simulink model "basicModel_old"  (R2017b)
settings: Solver=ode3  StartTime=0.0  StopTime=40  FixedStep=0.01  RelTol=1e-3  EnableMultiTasking=on
InitFcn:
  | clear;
  | clc;
  | Iniparameters
StopFcn:
  | simplot
values from neighbouring files (symbols this model uses):
  aaa = inv([kf kf kf kf;0 -kf 0 kf;-kf 0 kf 0;-km km -km km])    [Iniparameters.m]
  g = 9.8    [Iniparameters.m]
  Ixx = 19.688e-3    (= 0.019688)    [Iniparameters.m]
  Iyy = 19.688e-3    (= 0.019688)    [Iniparameters.m]
  Izz = 3.938e-2    (= 0.03938)    [Iniparameters.m]
  kdphi = 8    [Iniparameters.m]
  kdpsai = 8    [Iniparameters.m]
  kdtheta = kdphi    (= 8)    [Iniparameters.m]
  kdx = 0.55    [Iniparameters.m]
  kdy = 2.0    (= 2)    [Iniparameters.m]
  kdz = 2.4    [Iniparameters.m]
  kf = 3.13e-5    (= 3.13e-05)    [Iniparameters.m]
  kix = 0.001    [Iniparameters.m]
  kiy = 0.001    [Iniparameters.m]
  kiz = 0.001    [Iniparameters.m]
  km = 7.5e-7    (= 7.5e-07)    [Iniparameters.m]
  kpphi = 25    [Iniparameters.m]
  kppsai = 23    [Iniparameters.m]
  kptheta = kpphi    (= 25)    [Iniparameters.m]
  kpx = 0.75    [Iniparameters.m]
  kpy = 1.4    [Iniparameters.m]
  kpz = 2.9    [Iniparameters.m]
  L = 0.25    [Iniparameters.m]
  m = 0.75    [Iniparameters.m]
  wh = sqrt(m*g/(4*kf))    [Iniparameters.m]
  xf = 5    [Iniparameters.m]
  yaw = 0    [Iniparameters.m]
  yf = 5    [Iniparameters.m]
  zf = 5    [Iniparameters.m]
libraries: aerolibconvert2 x4
settings Model: Creator=KingBoy  LastModifiedBy=KingBoy
settings DataIOCC: LimitDataPoints=on  SaveFormat=Array
settings OptimizationCC: LifeSpan=inf
settings DebuggingCC: UnderspecifiedInitializationDetection=Classic  MergeDetectMultiDrivingBlocksExec=none  SolverPrmCheckMsg=warning  AllowSymbolicDim=off  SFUnexpectedBacktrackingDiag=warning  SFNoUnconditionalDefaultTransitionDiag=warning  SFExecutionAtInitializationDiag=none
settings HardwareCC: ProdBitPerPointer=32  ProdBitPerSizeT=32  ProdBitPerPtrDiffT=32  ProdLargestAtomicFloat=None  ProdIntDivRoundTo=Undefined  ProdEndianess=Unspecified  ProdWordSize=32  ProdHWDeviceType=32-bit Generic
settings ModelReferenceCC: PropagateSignalLabelsOutOfModel=off
settings CodeAppCC: StateflowObjectComments=on
settings GRTTargetCC: TargetLangStandard=C89/C90 (ANSI)  GeneratePreprocessorConditionals=Disable all
settings ConfigComp: CovMetricSettings=dw  CovHtmlReporting=on  CovSaveCumulativeToWorkspaceVar=on  CovSaveSingleToWorkspaceVar=on  CovExternalEMLEnable=off  CovSFcnEnable=off

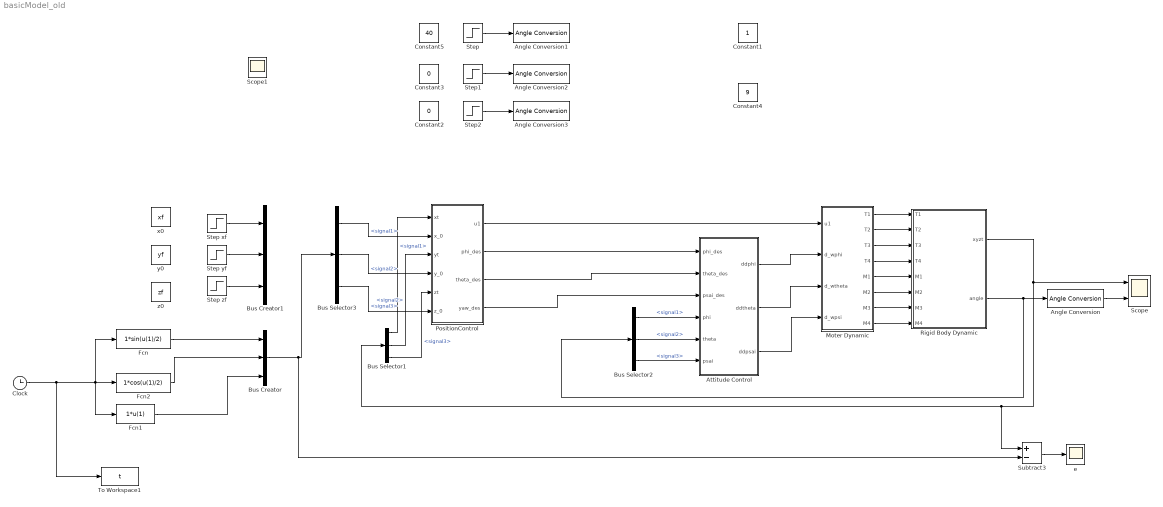
== system basicModel_old ==
  Angle Conversion : aerolibconvert2/Angle Conversion  IU=rad  OU=deg
  Angle Conversion1 : aerolibconvert2/Angle Conversion  IU=deg  OU=rad
  Angle Conversion2 : aerolibconvert2/Angle Conversion  IU=deg  OU=rad
  Angle Conversion3 : aerolibconvert2/Angle Conversion  IU=deg  OU=rad
  Attitude Control : Subsystem
  Bus Creator : BusCreator  Inputs=3
  Bus Creator1 : BusCreator  Inputs=3
  Bus Selector1 : BusSelector  OutputSignals=signal1,signal2,signal3
  Bus Selector2 : BusSelector  OutputSignals=signal1,signal2,signal3
  Bus Selector3 : BusSelector  OutputSignals=signal1,signal2,signal3
  Clock : Clock
  Constant1 : Constant
  Constant2 : Constant  Value=0
  Constant3 : Constant  Value=0
  Constant4 : Constant  Value=9
  Constant5 : Constant  Value=40
  Fcn : Fcn  Expr=1*sin(u(1)/2)
  Fcn1 : Fcn  Expr=1*u(1)
  Fcn2 : Fcn  Expr=1*cos(u(1)/2)
  Moter Dynamic : Subsystem
  PositionControl : Subsystem
  Rigid Body Dynamic : Subsystem
  Scope : Scope  NumInputPorts=2
  Scope1 : Scope
  Step : Step  After=xf  SampleTime=0
  Step xf : Step  After=xf  SampleTime=0
  Step yf : Step  After=yf  SampleTime=0
  Step zf : Step  After=zf  SampleTime=0
  Step1 : Step  After=yf  SampleTime=0
  Step2 : Step  After=zf  SampleTime=0
  Subtract3 : Sum  Inputs=+-
  To Workspace1 : ToWorkspace  VariableName=t  SampleTime=-1
      settings: Save2DSignal=2-D array (concatenate along first dimension)
  e : Scope
  x0 : Constant  Value=xf
  y0 : Constant  Value=yf
  z0 : Constant  Value=zf
  wires:
  Moter Dynamic/1(T1) -> Rigid Body Dynamic/1(T1)
  Moter Dynamic/2(T2) -> Rigid Body Dynamic/2(T2)
  Moter Dynamic/3(T3) -> Rigid Body Dynamic/3(T3)
  Moter Dynamic/4(T4) -> Rigid Body Dynamic/4(T4)
  Moter Dynamic/5(M1) -> Rigid Body Dynamic/5(M1)
  Moter Dynamic/6(M2) -> Rigid Body Dynamic/6(M2)
  Moter Dynamic/7(M3) -> Rigid Body Dynamic/7(M3)
  Moter Dynamic/8(M4) -> Rigid Body Dynamic/8(M4)
  Rigid Body Dynamic/1(xyzt) -> Subtract3/1, Bus Selector1/1, Scope/1
  Bus Selector1/1 -> PositionControl/1(xt)  "<signal1>"
  Bus Selector1/2 -> PositionControl/3(yt)  "<signal2>"
  Bus Selector1/3 -> PositionControl/5(zt)  "<signal3>"
  Rigid Body Dynamic/2(angle) -> Angle Conversion/1, Bus Selector2/1
  Angle Conversion/1 -> Scope/2
  Clock/1 -> To Workspace1/1, Fcn1/1, Fcn/1, Fcn2/1
  Fcn/1 -> Bus Creator/1
  Fcn2/1 -> Bus Creator/2
  Fcn1/1 -> Bus Creator/3
  Subtract3/1 -> e/1
  Bus Selector3/1 -> PositionControl/2(x_0)  "<signal1>"
  Bus Selector3/2 -> PositionControl/4(y_0)  "<signal2>"
  Bus Selector3/3 -> PositionControl/6(z_0)  "<signal3>"
  Step/1 -> Angle Conversion1/1
  Step2/1 -> Angle Conversion3/1
  Step1/1 -> Angle Conversion2/1
  Step zf/1 -> Bus Creator1/3
  Step yf/1 -> Bus Creator1/2
  Step xf/1 -> Bus Creator1/1
  Bus Selector2/3 -> Attitude Control/6(psai)  "<signal3>"
  Bus Selector2/2 -> Attitude Control/5(theta)  "<signal2>"
  Bus Selector2/1 -> Attitude Control/4(phi)  "<signal1>"
  Attitude Control/3(ddpsai) -> Moter Dynamic/4(d_wpsi)
  Attitude Control/2(ddtheta) -> Moter Dynamic/3(d_wtheta)
  Attitude Control/1(ddphi) -> Moter Dynamic/2(d_wphi)
  PositionControl/1(u1) -> Moter Dynamic/1(u1)
  PositionControl/2(phi_des) -> Attitude Control/1(phi_des)
  PositionControl/3(theta_des) -> Attitude Control/2(theta_des)
  PositionControl/4(yaw_des) -> Attitude Control/3(psai_des)
  Bus Creator/1 -> Subtract3/2, Bus Selector3/1

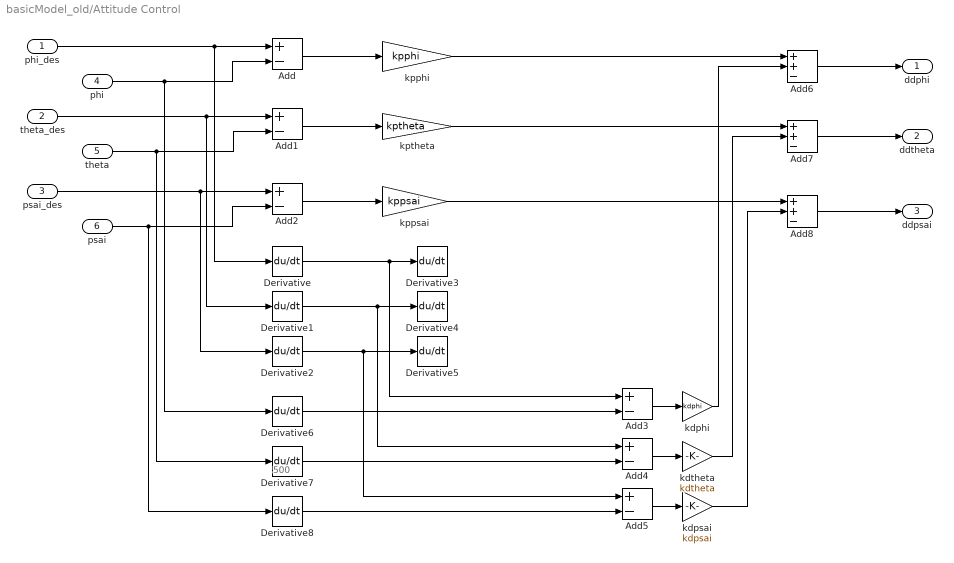
== system basicModel_old/Attitude Control ==
  note: 500
  phi_des : Inport
  theta_des : Inport  Port=2
  psai_des : Inport  Port=3
  phi : Inport  Port=4
  theta : Inport  Port=5
  psai : Inport  Port=6
  Add{,1..5} (6 alike) : Sum  Inputs=+-
  Add6 : Sum  Inputs=++-
  Add7 : Sum  Inputs=++-
  Add8 : Sum  Inputs=++-
  Derivative{,1..8} (9 alike) : Derivative  CoefficientInTFapproximation=500
  kdphi : Gain  Gain=kdphi
  kdpsai : Gain  Gain=kdpsai
  kdtheta : Gain  Gain=kdtheta
  kpphi : Gain  Gain=kpphi
  kppsai : Gain  Gain=kppsai
  kptheta : Gain  Gain=kptheta
  ddphi : Outport
  ddtheta : Outport  Port=2
  ddpsai : Outport  Port=3
  wires:
  phi_des/1 -> Add/1, Derivative/1
  phi/1 -> Derivative6/1, Add/2
  Add/1 -> kpphi/1
  theta_des/1 -> Derivative1/1, Add1/1
  theta/1 -> Derivative7/1, Add1/2
  Add1/1 -> kptheta/1
  Add2/1 -> kppsai/1
  psai_des/1 -> Derivative2/1, Add2/1
  psai/1 -> Derivative8/1, Add2/2
  Add3/1 -> kdphi/1
  Add4/1 -> kdtheta/1
  Add5/1 -> kdpsai/1
  kpphi/1 -> Add6/1
  kdphi/1 -> Add6/2
  kptheta/1 -> Add7/1
  kdtheta/1 -> Add7/2
  kppsai/1 -> Add8/1
  kdpsai/1 -> Add8/2
  Add6/1 -> ddphi/1
  Add7/1 -> ddtheta/1
  Add8/1 -> ddpsai/1
  Derivative/1 -> Add3/1, Derivative3/1
  Derivative1/1 -> Add4/1, Derivative4/1
  Derivative2/1 -> Add5/1, Derivative5/1
  Derivative6/1 -> Add3/2
  Derivative7/1 -> Add4/2
  Derivative8/1 -> Add5/2

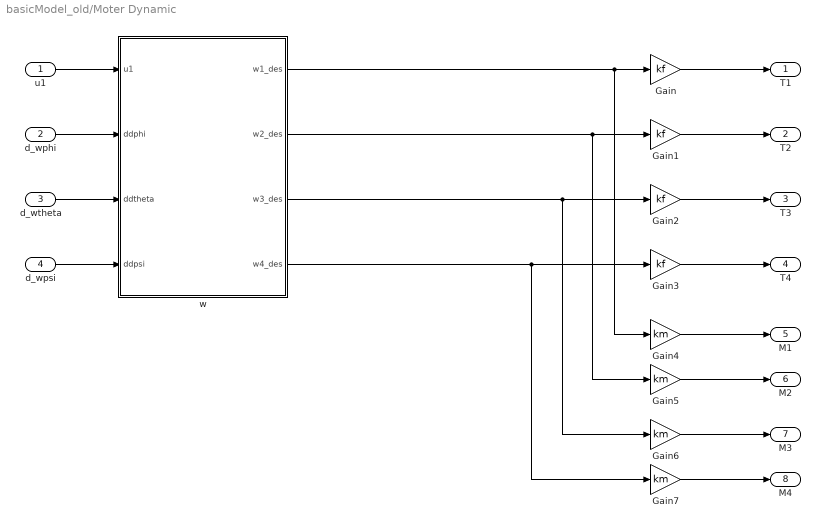
== system basicModel_old/Moter Dynamic ==
  u1 : Inport
  d_wphi : Inport  Port=2
  d_wtheta : Inport  Port=3
  d_wpsi : Inport  Port=4
  Gain{,1..3} (4 alike) : Gain  Gain=kf
  Gain{4..7} (4 alike) : Gain  Gain=km
  w : Subsystem
  T1 : Outport
  T2 : Outport  Port=2
  T3 : Outport  Port=3
  T4 : Outport  Port=4
  M1 : Outport  Port=5
  M2 : Outport  Port=6
  M3 : Outport  Port=7
  M4 : Outport  Port=8
  wires:
  u1/1 -> w/1(u1)
  d_wphi/1 -> w/2(ddphi)
  d_wtheta/1 -> w/3(ddtheta)
  d_wpsi/1 -> w/4(ddpsi)
  Gain/1 -> T1/1
  Gain1/1 -> T2/1
  Gain2/1 -> T3/1
  Gain3/1 -> T4/1
  Gain4/1 -> M1/1
  Gain5/1 -> M2/1
  Gain6/1 -> M3/1
  Gain7/1 -> M4/1
  w/4(w4_des) -> Gain7/1, Gain3/1
  w/3(w3_des) -> Gain6/1, Gain2/1
  w/2(w2_des) -> Gain5/1, Gain1/1
  w/1(w1_des) -> Gain4/1, Gain/1

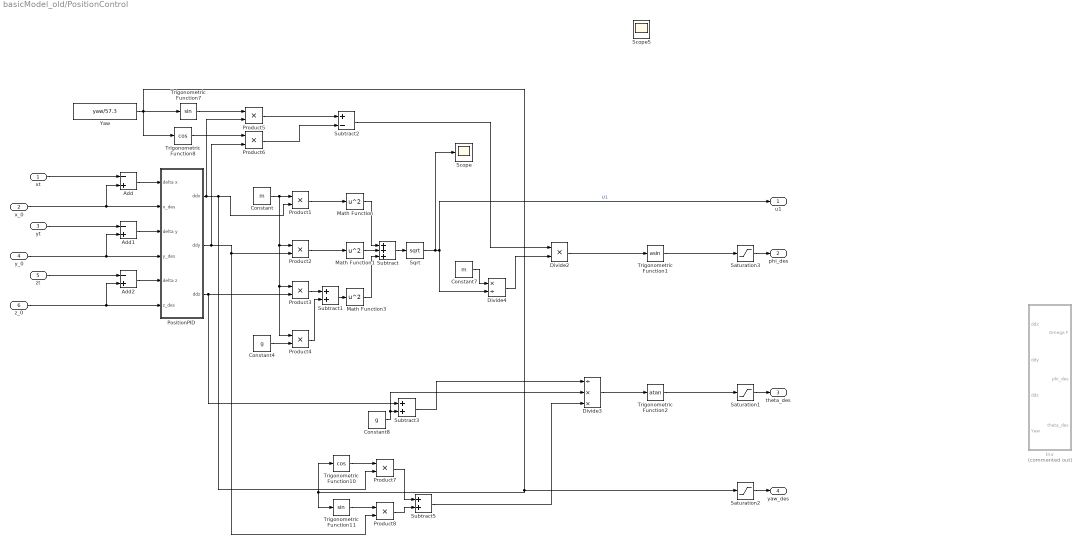
== system basicModel_old/PositionControl ==
  xt : Inport
  x_0 : Inport  Port=2
  yt : Inport  Port=3
  y_0 : Inport  Port=4
  zt : Inport  Port=5
  z_0 : Inport  Port=6
  Add : Sum  Inputs=-+
  Add1 : Sum  Inputs=-+
  Add2 : Sum  Inputs=-+
  Constant : Constant  Value=m
  Constant4 : Constant  Value=g
  Constant7 : Constant  Value=m
  Constant8 : Constant  Value=g
  Divide2 : Product  Inputs=**
  Divide3 : Product  Inputs=/**
  Divide4 : Product  Inputs=*/
  Inv : Subsystem  Commented=on
  Math Function : Math  Operator=square  SaturateOnIntegerOverflow=on
  Math Function1 : Math  Operator=square  SaturateOnIntegerOverflow=on
  Math Function3 : Math  Operator=square  SaturateOnIntegerOverflow=on
  PositionPID : Subsystem
  Product{1..8} (8 alike) : Product
  Saturation1 : Saturate  UpperLimit=90/57.3  LowerLimit=-90/57.3
  Saturation2 : Saturate  UpperLimit=90/57.3  LowerLimit=-90/57.3
  Saturation3 : Saturate  UpperLimit=90/57.3  LowerLimit=-90/57.3
  Scope : Scope
  Scope5 : Scope
  Sqrt : Sqrt  SaturateOnIntegerOverflow=on
  Subtract : Sum  Inputs=+++
  Subtract1 : Sum
  Subtract2 : Sum  Inputs=+-
  Subtract3 : Sum
  Subtract5 : Sum
  Trigonometric Function1 : Trigonometry  Operator=asin
  Trigonometric Function10 : Trigonometry  Operator=cos
  Trigonometric Function11 : Trigonometry
  Trigonometric Function2 : Trigonometry  Operator=atan
  Trigonometric Function7 : Trigonometry
  Trigonometric Function8 : Trigonometry  Operator=cos
  Yaw : Constant  Value=yaw/57.3
  u1 : Outport
  phi_des : Outport  Port=2
  theta_des : Outport  Port=3
  yaw_des : Outport  Port=4
  wires:
  xt/1 -> Add/1
  x_0/1 -> Add/2, PositionPID/2(x_des)
  Add/1 -> PositionPID/1(delta x)
  yt/1 -> Add1/1
  y_0/1 -> Add1/2, PositionPID/4(y_des)
  Add1/1 -> PositionPID/3(delta y)
  zt/1 -> Add2/1
  z_0/1 -> Add2/2, PositionPID/6(z_des)
  Add2/1 -> PositionPID/5(delta z)
  Product1/1 -> Math Function/1
  Constant/1 -> Product4/1, Product3/1, Product2/1, Product1/1
  Product2/1 -> Math Function1/1
  PositionPID/2(ddy) -> Product6/2, Product2/2, Product8/2
  Subtract/1 -> Sqrt/1
  Constant4/1 -> Product4/2
  Product3/1 -> Subtract1/1
  Product4/1 -> Subtract1/2
  Subtract1/1 -> Math Function3/1
  Math Function1/1 -> Subtract/2
  Math Function/1 -> Subtract/1
  Math Function3/1 -> Subtract/3
  Sqrt/1 -> Scope/1, Divide4/2, u1/1  "U1"
  PositionPID/3(ddz) -> Subtract3/1, Product3/2
  Product5/1 -> Subtract2/1
  Product6/1 -> Subtract2/2
  Subtract2/1 -> Divide2/1
  Divide3/1 -> Trigonometric Function2/1
  Constant7/1 -> Divide4/1
  Divide4/1 -> Divide2/2
  Constant8/1 -> Divide3/2, Subtract3/2
  Trigonometric Function2/1 -> Saturation1/1
  Trigonometric Function1/1 -> Saturation3/1
  Divide2/1 -> Trigonometric Function1/1
  PositionPID/1(ddx) -> Product1/2, Product7/2, Product5/2
  Trigonometric Function7/1 -> Product5/1
  Trigonometric Function8/1 -> Product6/1
  Yaw/1 -> Trigonometric Function10/1, Trigonometric Function11/1, Saturation2/1, Trigonometric Function8/1, Trigonometric Function7/1
  Trigonometric Function10/1 -> Product7/1
  Trigonometric Function11/1 -> Product8/1
  Product7/1 -> Subtract5/1
  Product8/1 -> Subtract5/2
  Subtract5/1 -> Divide3/3
  Subtract3/1 -> Divide3/1
  Saturation3/1 -> phi_des/1
  Saturation1/1 -> theta_des/1
  Saturation2/1 -> yaw_des/1

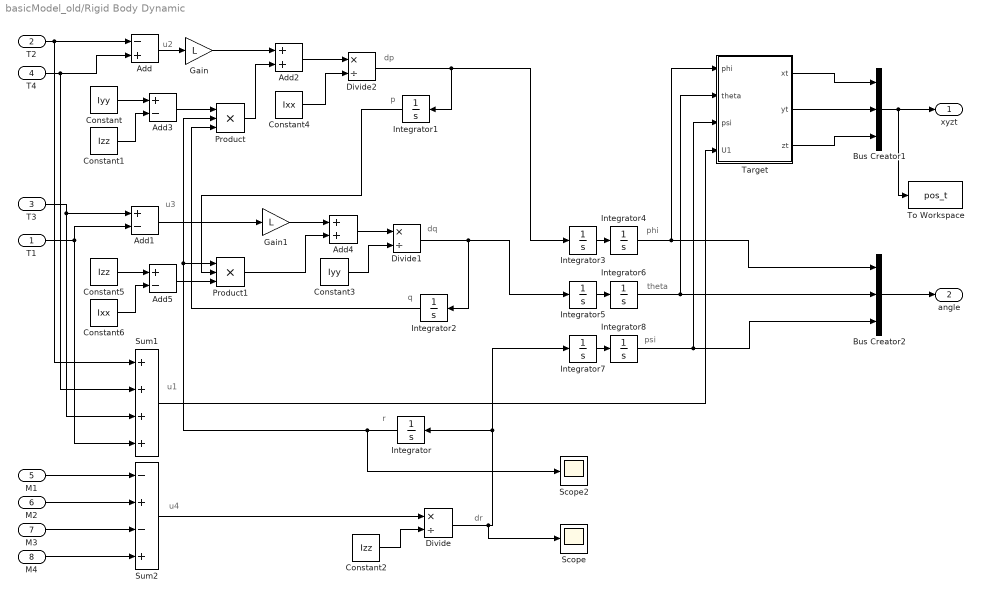
== system basicModel_old/Rigid Body Dynamic ==
  note: psi
  note: theta
  note: phi
  note: p
  note: q
  note: dq
  note: dp
  note: u4
  note: u3
  note: u2
  note: u1
  note: r
  note: dr
  T1 : Inport
  T2 : Inport  Port=2
  T3 : Inport  Port=3
  T4 : Inport  Port=4
  M1 : Inport  Port=5
  M2 : Inport  Port=6
  M3 : Inport  Port=7
  M4 : Inport  Port=8
  Add : Sum  Inputs=-+
  Add1 : Sum  Inputs=+-
  Add2 : Sum
  Add3 : Sum  Inputs=+-
  Add4 : Sum
  Add5 : Sum  Inputs=+-
  Bus Creator1 : BusCreator  Inputs=3
  Bus Creator2 : BusCreator  Inputs=3
  Constant : Constant  Value=Iyy
  Constant1 : Constant  Value=Izz
  Constant2 : Constant  Value=Izz
  Constant3 : Constant  Value=Iyy
  Constant4 : Constant  Value=Ixx
  Constant5 : Constant  Value=Izz
  Constant6 : Constant  Value=Ixx
  Divide : Product  Inputs=*/
  Divide1 : Product  Inputs=*/
  Divide2 : Product  Inputs=*/
  Gain : Gain  Gain=L
  Gain1 : Gain  Gain=L
  Integrator : Integrator  UpperSaturationLimit=50  LowerSaturationLimit=-50
  Integrator{1..8} (8 alike) : Integrator
  Product : Product  Inputs=3
  Product1 : Product  Inputs=3
  Scope : Scope
  Scope2 : Scope
  Sum1 : Sum  Inputs=++++
  Sum2 : Sum  Inputs=-+-+
  Target : Subsystem
  To Workspace : ToWorkspace  VariableName=pos_t  SampleTime=-1
      settings: Save2DSignal=2-D array (concatenate along first dimension)
  xyzt : Outport
  angle : Outport  Port=2
  wires:
  T2/1 -> Add/1, Sum1/1
  T4/1 -> Add/2, Sum1/2
  Add/1 -> Gain/1
  Add1/1 -> Gain1/1
  Gain/1 -> Add2/1
  Constant/1 -> Add3/1
  Constant1/1 -> Add3/2
  Add3/1 -> Product/1
  Product/1 -> Add2/2
  M1/1 -> Sum2/1
  M2/1 -> Sum2/2
  M3/1 -> Sum2/3
  M4/1 -> Sum2/4
  Constant2/1 -> Divide/2
  Divide/1 -> Scope/1, Integrator/1, Integrator7/1
  Integrator/1 -> Scope2/1, Product1/1, Product/2
  Gain1/1 -> Add4/1
  T3/1 -> Add1/1, Sum1/3
  T1/1 -> Add1/2, Sum1/4
  Add4/1 -> Divide1/1
  Constant3/1 -> Divide1/2
  Sum1/1 -> Target/4(U1)
  Add2/1 -> Divide2/1
  Constant4/1 -> Divide2/2
  Divide2/1 -> Integrator1/1, Integrator3/1
  Divide1/1 -> Integrator5/1, Integrator2/1
  Integrator2/1 -> Product/3
  Constant5/1 -> Add5/1
  Constant6/1 -> Add5/2
  Add5/1 -> Product1/3
  Product1/1 -> Add4/2
  Integrator1/1 -> Product1/2
  Integrator4/1 -> Bus Creator2/1, Target/1(phi)
  Integrator6/1 -> Bus Creator2/2, Target/2(theta)
  Integrator8/1 -> Target/3(psi), Bus Creator2/3
  Bus Creator2/1 -> angle/1
  Target/1(xt) -> Bus Creator1/1
  Target/2(yt) -> Bus Creator1/2
  Target/3(zt) -> Bus Creator1/3
  Integrator3/1 -> Integrator4/1
  Integrator5/1 -> Integrator6/1
  Integrator7/1 -> Integrator8/1
  Sum2/1 -> Divide/1
  Bus Creator1/1 -> xyzt/1, To Workspace/1

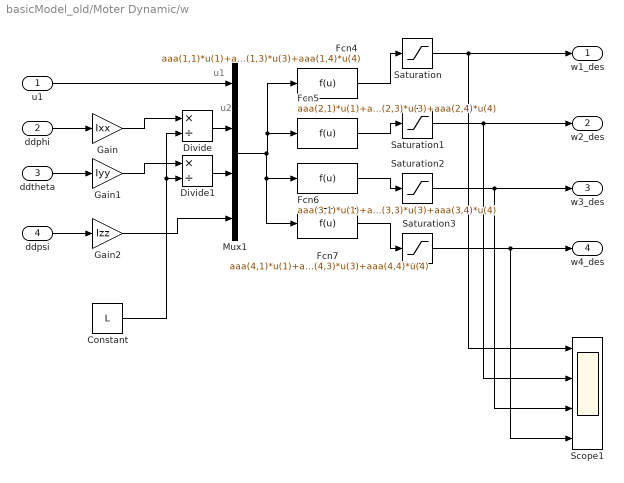
== system basicModel_old/Moter Dynamic/w ==
  note: u2
  note: u1
  u1 : Inport
  ddphi : Inport  Port=2
  ddtheta : Inport  Port=3
  ddpsi : Inport  Port=4
  Constant : Constant  Value=L
  Divide : Product  Inputs=*/
  Divide1 : Product  Inputs=*/
  Fcn4 : Fcn  Expr=aaa(1,1)*u(1)+aaa(1,2)*u(2)+aaa(1,3)*u(3)+aaa(1,4)*u(4)
  Fcn5 : Fcn  Expr=aaa(2,1)*u(1)+aaa(2,2)*u(2)+aaa(2,3)*u(3)+aaa(2,4)*u(4)
  Fcn6 : Fcn  Expr=aaa(3,1)*u(1)+aaa(3,2)*u(2)+aaa(3,3)*u(3)+aaa(3,4)*u(4)
  Fcn7 : Fcn  Expr=aaa(4,1)*u(1)+aaa(4,2)*u(2)+aaa(4,3)*u(3)+aaa(4,4)*u(4)
  Gain : Gain  Gain=Ixx
  Gain1 : Gain  Gain=Iyy
  Gain2 : Gain  Gain=Izz
  Mux1 : Mux
  Saturation{,1..3} (4 alike) : Saturate  UpperLimit=6000^2  LowerLimit=0
  Scope1 : Scope  NumInputPorts=4
  w1_des : Outport
  w2_des : Outport  Port=2
  w3_des : Outport  Port=3
  w4_des : Outport  Port=4
  wires:
  u1/1 -> Mux1/1
  ddphi/1 -> Gain/1
  ddpsi/1 -> Gain2/1
  ddtheta/1 -> Gain1/1
  Mux1/1 -> Fcn7/1, Fcn6/1, Fcn5/1, Fcn4/1
  Fcn4/1 -> Saturation/1
  Fcn6/1 -> Saturation2/1
  Fcn7/1 -> Saturation3/1
  Saturation/1 -> Scope1/1, w1_des/1
  Saturation1/1 -> Scope1/2, w2_des/1
  Saturation2/1 -> Scope1/3, w3_des/1
  Saturation3/1 -> Scope1/4, w4_des/1
  Divide/1 -> Mux1/2
  Gain/1 -> Divide/1
  Constant/1 -> Divide/2, Divide1/2
  Divide1/1 -> Mux1/3
  Gain2/1 -> Mux1/4
  Gain1/1 -> Divide1/1
  Fcn5/1 -> Saturation1/1

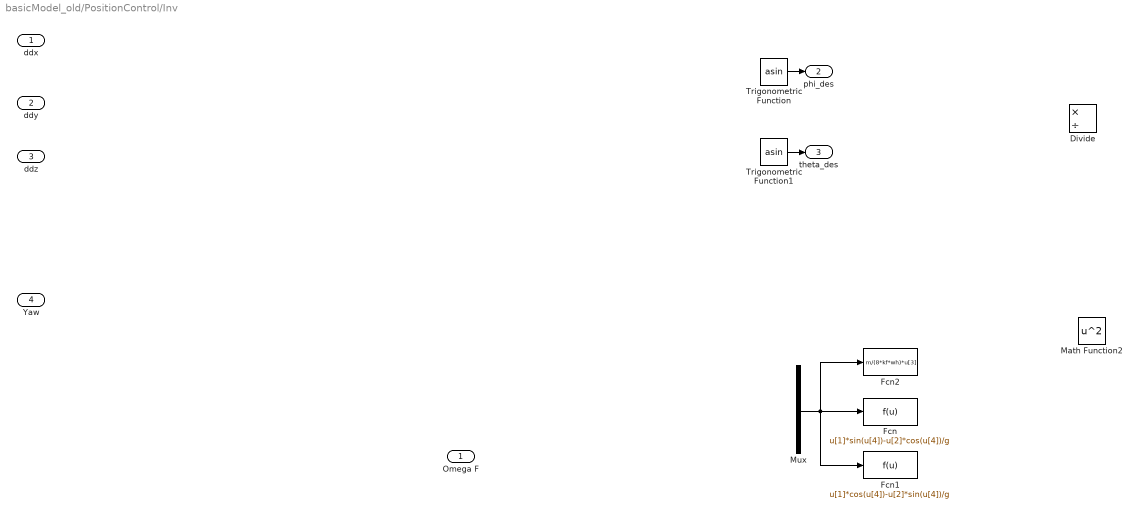
== system basicModel_old/PositionControl/Inv ==
  ddx : Inport
  ddy : Inport  Port=2
  ddz : Inport  Port=3
  Yaw : Inport  Port=4
  Divide : Product  Inputs=*/
  Fcn : Fcn  Expr=u[1]*sin(u[4])-u[2]*cos(u[4])/g
  Fcn1 : Fcn  Expr=u[1]*cos(u[4])-u[2]*sin(u[4])/g
  Fcn2 : Fcn  Expr=m/(8*kf*wh)*u[3]
  Math Function2 : Math  Operator=square  SaturateOnIntegerOverflow=on
  Mux : Mux
  Trigonometric Function : Trigonometry  Operator=asin
  Trigonometric Function1 : Trigonometry  Operator=asin
  Omega F : Outport
  phi_des : Outport  Port=2
  theta_des : Outport  Port=3
  wires:
  Mux/1 -> Fcn1/1, Fcn/1, Fcn2/1
  Trigonometric Function/1 -> phi_des/1
  Trigonometric Function1/1 -> theta_des/1

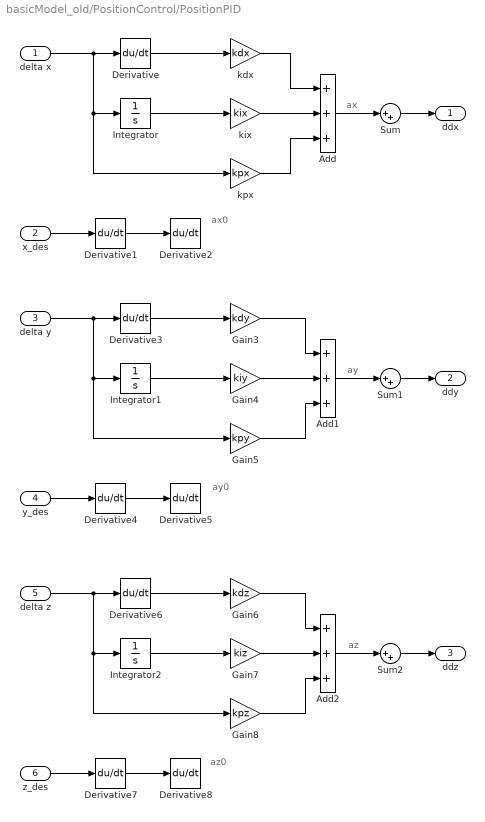
== system basicModel_old/PositionControl/PositionPID ==
  note: az
  note: ay
  note: ax
  note: az0
  note: ay0
  note: ax0
  delta x : Inport
  x_des : Inport  Port=2
  delta y : Inport  Port=3
  y_des : Inport  Port=4
  delta z : Inport  Port=5
  z_des : Inport  Port=6
  Add : Sum  Inputs=+++
  Add1 : Sum  Inputs=+++
  Add2 : Sum  Inputs=+++
  Derivative{,1..5,7..8} (8 alike) : Derivative  CoefficientInTFapproximation=500
  Derivative6 : Derivative
  Gain3 : Gain  Gain=kdy
  Gain4 : Gain  Gain=kiy
  Gain5 : Gain  Gain=kpy
  Gain6 : Gain  Gain=kdz
  Gain7 : Gain  Gain=kiz
  Gain8 : Gain  Gain=kpz
  Integrator : Integrator
  Integrator1 : Integrator
  Integrator2 : Integrator
  Sum : Sum  Inputs=|++
  Sum1 : Sum  Inputs=|++
  Sum2 : Sum  Inputs=|++
  kdx : Gain  Gain=kdx
  kix : Gain  Gain=kix
  kpx : Gain  Gain=kpx
  ddx : Outport
  ddy : Outport  Port=2
  ddz : Outport  Port=3
  wires:
  delta x/1 -> kpx/1, Integrator/1, Derivative/1
  Derivative/1 -> kdx/1
  kdx/1 -> Add/1
  Integrator/1 -> kix/1
  kix/1 -> Add/2
  kpx/1 -> Add/3
  Add/1 -> Sum/1
  Derivative1/1 -> Derivative2/1
  x_des/1 -> Derivative1/1
  Sum/1 -> ddx/1
  delta y/1 -> Gain5/1, Integrator1/1, Derivative3/1
  Derivative3/1 -> Gain3/1
  Gain3/1 -> Add1/1
  Integrator1/1 -> Gain4/1
  Gain4/1 -> Add1/2
  Gain5/1 -> Add1/3
  Add1/1 -> Sum1/1
  Derivative4/1 -> Derivative5/1
  y_des/1 -> Derivative4/1
  Sum1/1 -> ddy/1
  delta z/1 -> Gain8/1, Integrator2/1, Derivative6/1
  Derivative6/1 -> Gain6/1
  Gain6/1 -> Add2/1
  Integrator2/1 -> Gain7/1
  Gain7/1 -> Add2/2
  Gain8/1 -> Add2/3
  Add2/1 -> Sum2/1
  Derivative7/1 -> Derivative8/1
  z_des/1 -> Derivative7/1
  Sum2/1 -> ddz/1

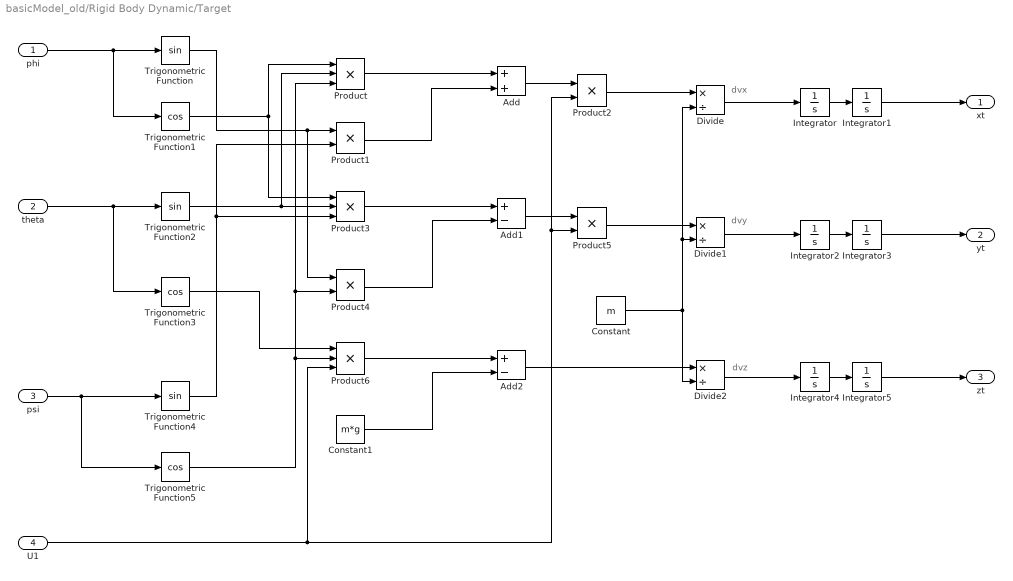
== system basicModel_old/Rigid Body Dynamic/Target ==
  note: dvz
  note: dvy
  note: dvx
  phi : Inport
  theta : Inport  Port=2
  psi : Inport  Port=3
  U1 : Inport  Port=4
  Add : Sum
  Add1 : Sum  Inputs=+-
  Add2 : Sum  Inputs=+-
  Constant : Constant  Value=m
  Constant1 : Constant  Value=m*g
  Divide : Product  Inputs=*/
  Divide1 : Product  Inputs=*/
  Divide2 : Product  Inputs=*/
  Integrator{,1..5} (6 alike) : Integrator
  Product : Product  Inputs=3
  Product{1..2,4..5} (4 alike) : Product
  Product3 : Product  Inputs=3
  Product6 : Product  Inputs=3
  Trigonometric Function : Trigonometry
  Trigonometric Function1 : Trigonometry  Operator=cos
  Trigonometric Function2 : Trigonometry
  Trigonometric Function3 : Trigonometry  Operator=cos
  Trigonometric Function4 : Trigonometry
  Trigonometric Function5 : Trigonometry  Operator=cos
  xt : Outport
  yt : Outport  Port=2
  zt : Outport  Port=3
  wires:
  phi/1 -> Trigonometric Function1/1, Trigonometric Function/1
  theta/1 -> Trigonometric Function3/1, Trigonometric Function2/1
  Integrator/1 -> Integrator1/1
  Integrator2/1 -> Integrator3/1
  Integrator4/1 -> Integrator5/1
  Integrator5/1 -> zt/1
  Integrator3/1 -> yt/1
  Integrator1/1 -> xt/1
  Trigonometric Function1/1 -> Product3/1, Product/1
  Trigonometric Function2/1 -> Product3/2, Product/2
  Trigonometric Function5/1 -> Product6/2, Product4/2, Product/3
  Product/1 -> Add/1
  Divide/1 -> Integrator/1
  Trigonometric Function/1 -> Product4/1, Product1/1
  Trigonometric Function4/1 -> Product3/3, Product1/2
  Product1/1 -> Add/2
  Add/1 -> Product2/1
  U1/1 -> Product6/3, Product5/2, Product2/2
  Product3/1 -> Add1/1
  Product4/1 -> Add1/2
  Add1/1 -> Product5/1
  Divide1/1 -> Integrator2/1
  Trigonometric Function3/1 -> Product6/1
  Divide2/1 -> Integrator4/1
  Constant1/1 -> Add2/2
  Product6/1 -> Add2/1
  Constant/1 -> Divide2/2, Divide/2, Divide1/2
  Product2/1 -> Divide/1
  Product5/1 -> Divide1/1
  Add2/1 -> Divide2/1
  psi/1 -> Trigonometric Function5/1, Trigonometric Function4/1
